simulink model "AFS_Master"  (R2020b)
settings: configuration reference "VLS_Standard_Configuration" (kept outside this file)
undefined symbols (not defined in the file): C_AFS_SpeedThrAct
libraries: AFS_MasterFeature x2
settings Model: DataDictionary=AFS_Master_Model.sldd  Creator=mmoufakk  LastModifiedBy=mtarek-a
settings ConfigSetRef: SourceName=VLS_Standard_Configuration

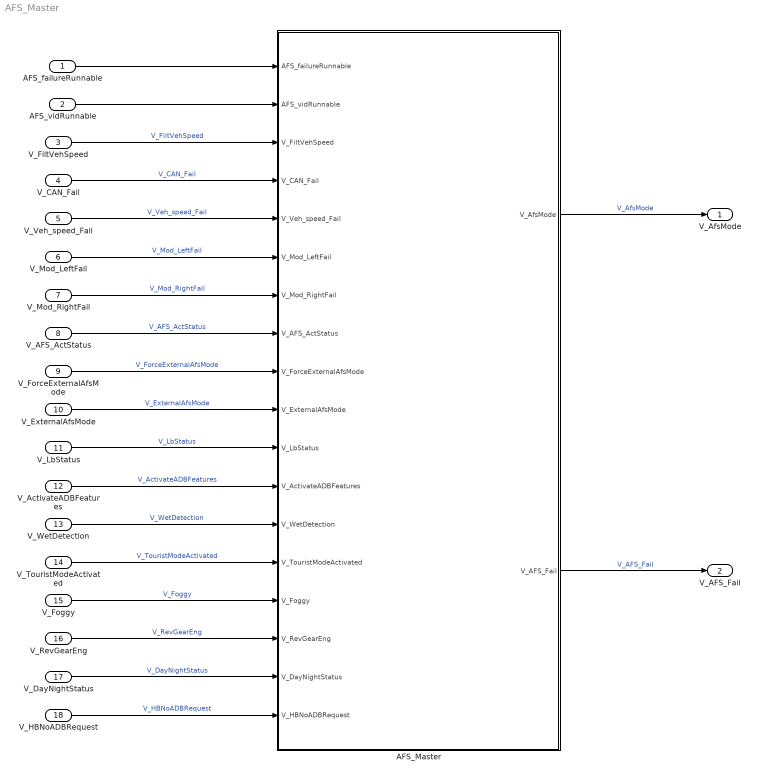
== system AFS_Master ==
  AFS_failureRunnable : Inport  OutputFunctionCall=on
  AFS_vidRunnable : Inport  Port=2  OutputFunctionCall=on
  V_FiltVehSpeed : Inport  Port=3
  V_CAN_Fail : Inport  Port=4
  V_Veh_speed_Fail : Inport  Port=5
  V_Mod_LeftFail : Inport  Port=6
  V_Mod_RightFail : Inport  Port=7
  V_AFS_ActStatus : Inport  Port=8
  V_ForceExternalAfsMode : Inport  Port=9
  V_ExternalAfsMode : Inport  Port=10
  V_LbStatus : Inport  Port=11
  V_ActivateADBFeatures : Inport  Port=12
  V_WetDetection : Inport  Port=13
  V_TouristModeActivated : Inport  Port=14
  V_Foggy : Inport  Port=15
  V_RevGearEng : Inport  Port=16
  V_DayNightStatus : Inport  Port=17
  V_HBNoADBRequest : Inport  Port=18
  AFS_Master : Subsystem  Description=AFS_Master
  V_AfsMode : Outport  PortDimensions=1
  V_AFS_Fail : Outport  Port=2  VectorParamsAs1DForOutWhenUnconnected=off
  wires:
  AFS_Master/1(V_AfsMode) -> V_AfsMode/1  "V_AfsMode"
  AFS_Master/2(V_AFS_Fail) -> V_AFS_Fail/1  "V_AFS_Fail"
  AFS_failureRunnable/1 -> AFS_Master/1(AFS_failureRunnable)
  AFS_vidRunnable/1 -> AFS_Master/2(AFS_vidRunnable)
  V_CAN_Fail/1 -> AFS_Master/4(V_CAN_Fail)  "V_CAN_Fail"
  V_Veh_speed_Fail/1 -> AFS_Master/5(V_Veh_speed_Fail)  "V_Veh_speed_Fail"
  V_Mod_LeftFail/1 -> AFS_Master/6(V_Mod_LeftFail)  "V_Mod_LeftFail"
  V_FiltVehSpeed/1 -> AFS_Master/3(V_FiltVehSpeed)  "V_FiltVehSpeed"
  V_ActivateADBFeatures/1 -> AFS_Master/12(V_ActivateADBFeatures)  "V_ActivateADBFeatures"
  V_Mod_RightFail/1 -> AFS_Master/7(V_Mod_RightFail)  "V_Mod_RightFail"
  V_AFS_ActStatus/1 -> AFS_Master/8(V_AFS_ActStatus)  "V_AFS_ActStatus"
  V_LbStatus/1 -> AFS_Master/11(V_LbStatus)  "V_LbStatus"
  V_WetDetection/1 -> AFS_Master/13(V_WetDetection)  "V_WetDetection"
  V_TouristModeActivated/1 -> AFS_Master/14(V_TouristModeActivated)  "V_TouristModeActivated"
  V_Foggy/1 -> AFS_Master/15(V_Foggy)  "V_Foggy"
  V_RevGearEng/1 -> AFS_Master/16(V_RevGearEng)  "V_RevGearEng"
  V_DayNightStatus/1 -> AFS_Master/17(V_DayNightStatus)  "V_DayNightStatus"
  V_HBNoADBRequest/1 -> AFS_Master/18(V_HBNoADBRequest)  "V_HBNoADBRequest"
  V_ForceExternalAfsMode/1 -> AFS_Master/9(V_ForceExternalAfsMode)  "V_ForceExternalAfsMode"
  V_ExternalAfsMode/1 -> AFS_Master/10(V_ExternalAfsMode)  "V_ExternalAfsMode"

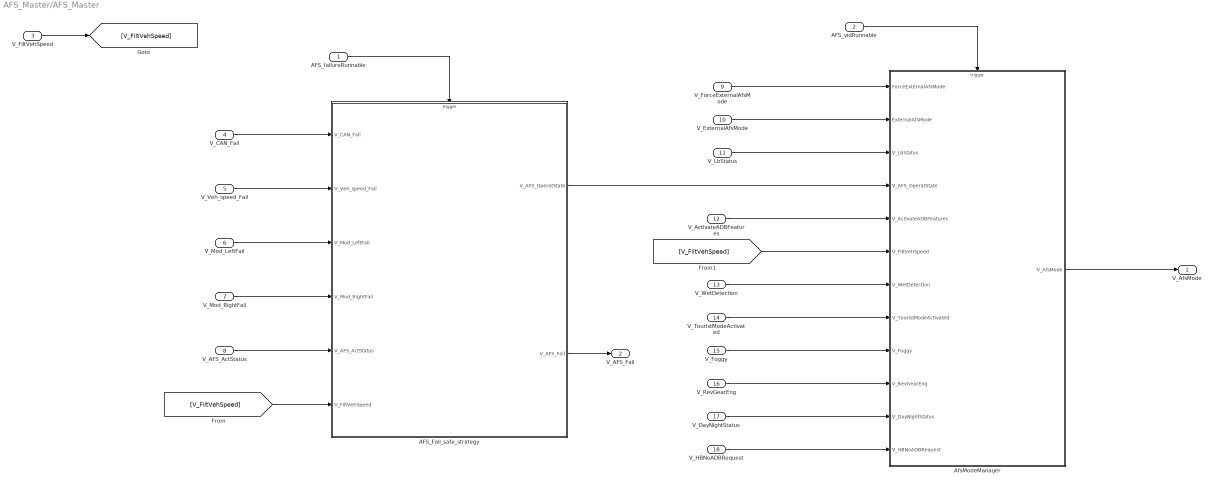
== system AFS_Master/AFS_Master ==
  AFS_failureRunnable : Inport  OutputFunctionCall=on
  AFS_vidRunnable : Inport  Port=2  OutputFunctionCall=on
  V_FiltVehSpeed : Inport  Port=3
  V_CAN_Fail : Inport  Port=4
  V_Veh_speed_Fail : Inport  Port=5
  V_Mod_LeftFail : Inport  Port=6
  V_Mod_RightFail : Inport  Port=7
  V_AFS_ActStatus : Inport  Port=8
  V_ForceExternalAfsMode : Inport  Port=9
  V_ExternalAfsMode : Inport  Port=10
  V_LbStatus : Inport  Port=11
  V_ActivateADBFeatures : Inport  Port=12
  V_WetDetection : Inport  Port=13
  V_TouristModeActivated : Inport  Port=14
  V_Foggy : Inport  Port=15
  V_RevGearEng : Inport  Port=16
  V_DayNightStatus : Inport  Port=17
  V_HBNoADBRequest : Inport  Port=18
  AFS_Fail_safe_strategy : Subsystem  Description=AFS_Fail_safe_strategy
  AfsModeManager : Subsystem  Description=AfsModeManager
  V_AfsMode : Outport  PortDimensions=1
  V_AFS_Fail : Outport  Port=2  VectorParamsAs1DForOutWhenUnconnected=off
  wires:
  V_HBNoADBRequest/1 -> AfsModeManager/12(V_HBNoADBRequest)
  V_DayNightStatus/1 -> AfsModeManager/11(V_DayNightStatus)
  AFS_Fail_safe_strategy/1(V_AFS_OperatState) -> AfsModeManager/4(V_AFS_OperatState)
  V_Mod_RightFail/1 -> AFS_Fail_safe_strategy/4(V_Mod_RightFail)
  V_Mod_LeftFail/1 -> AFS_Fail_safe_strategy/3(V_Mod_LeftFail)
  AFS_Fail_safe_strategy/2(V_AFS_Fail) -> V_AFS_Fail/1
  [V_FiltVehSpeed] -> AfsModeManager/6(V_FiltVehSpeed)
  [V_FiltVehSpeed] -> AFS_Fail_safe_strategy/6(V_FiltVehSpeed)
  V_FiltVehSpeed/1 -> [V_FiltVehSpeed]
  V_AFS_ActStatus/1 -> AFS_Fail_safe_strategy/5(V_AFS_ActStatus)
  AFS_failureRunnable/1 -> AFS_Fail_safe_strategy/Trigger
  V_Veh_speed_Fail/1 -> AFS_Fail_safe_strategy/2(V_Veh_speed_Fail)
  V_CAN_Fail/1 -> AFS_Fail_safe_strategy/1(V_CAN_Fail)
  AFS_vidRunnable/1 -> AfsModeManager/Trigger
  V_Foggy/1 -> AfsModeManager/9(V_Foggy)
  V_ForceExternalAfsMode/1 -> AfsModeManager/1(ForceExternalAfsMode)
  V_LbStatus/1 -> AfsModeManager/3(V_LbStatus)
  V_WetDetection/1 -> AfsModeManager/7(V_WetDetection)
  AfsModeManager/1(V_AfsMode) -> V_AfsMode/1
  V_RevGearEng/1 -> AfsModeManager/10(V_RevGearEng)
  V_ExternalAfsMode/1 -> AfsModeManager/2(ExternalAfsMode)
  V_ActivateADBFeatures/1 -> AfsModeManager/5(V_ActivateADBFeatures)
  V_TouristModeActivated/1 -> AfsModeManager/8(V_TouristModeActivated)

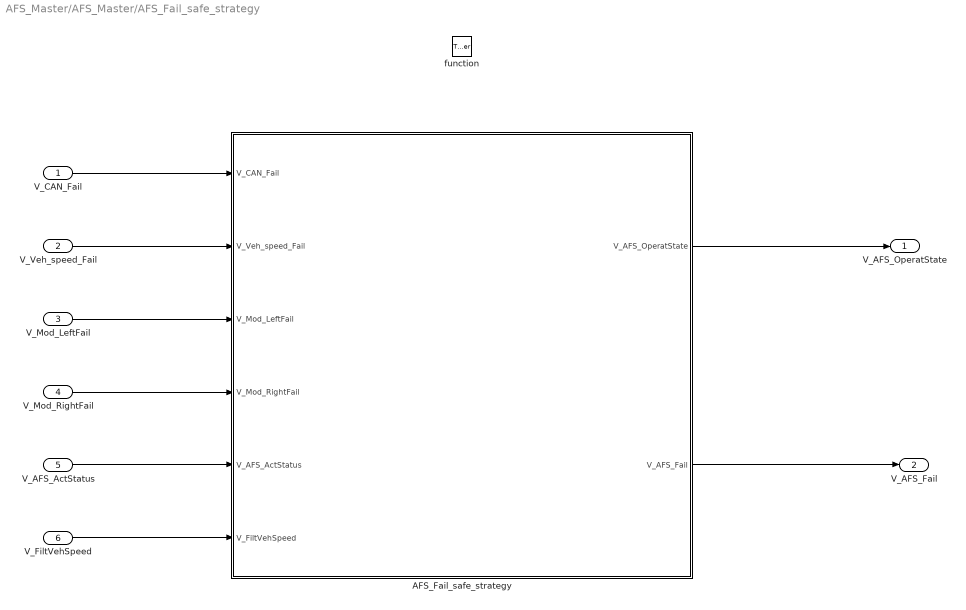
== system AFS_Master/AFS_Master/AFS_Fail_safe_strategy ==
  V_CAN_Fail : Inport
  V_Veh_speed_Fail : Inport  Port=2
  V_Mod_LeftFail : Inport  Port=3
  V_Mod_RightFail : Inport  Port=4
  V_AFS_ActStatus : Inport  Port=5
  V_FiltVehSpeed : Inport  Port=6
  function : TriggerPort  TriggerType=function-call  VariantControl=Variant
  AFS_Fail_safe_strategy : Subsystem  Description=AFS_Fail_safe_strategy
  V_AFS_OperatState : Outport  VectorParamsAs1DForOutWhenUnconnected=off
  V_AFS_Fail : Outport  Port=2  VectorParamsAs1DForOutWhenUnconnected=off
  wires:
  V_Veh_speed_Fail/1 -> AFS_Fail_safe_strategy/2(V_Veh_speed_Fail)
  V_CAN_Fail/1 -> AFS_Fail_safe_strategy/1(V_CAN_Fail)
  V_AFS_ActStatus/1 -> AFS_Fail_safe_strategy/5(V_AFS_ActStatus)
  V_Mod_LeftFail/1 -> AFS_Fail_safe_strategy/3(V_Mod_LeftFail)
  V_Mod_RightFail/1 -> AFS_Fail_safe_strategy/4(V_Mod_RightFail)
  AFS_Fail_safe_strategy/2(V_AFS_Fail) -> V_AFS_Fail/1
  AFS_Fail_safe_strategy/1(V_AFS_OperatState) -> V_AFS_OperatState/1
  V_FiltVehSpeed/1 -> AFS_Fail_safe_strategy/6(V_FiltVehSpeed)

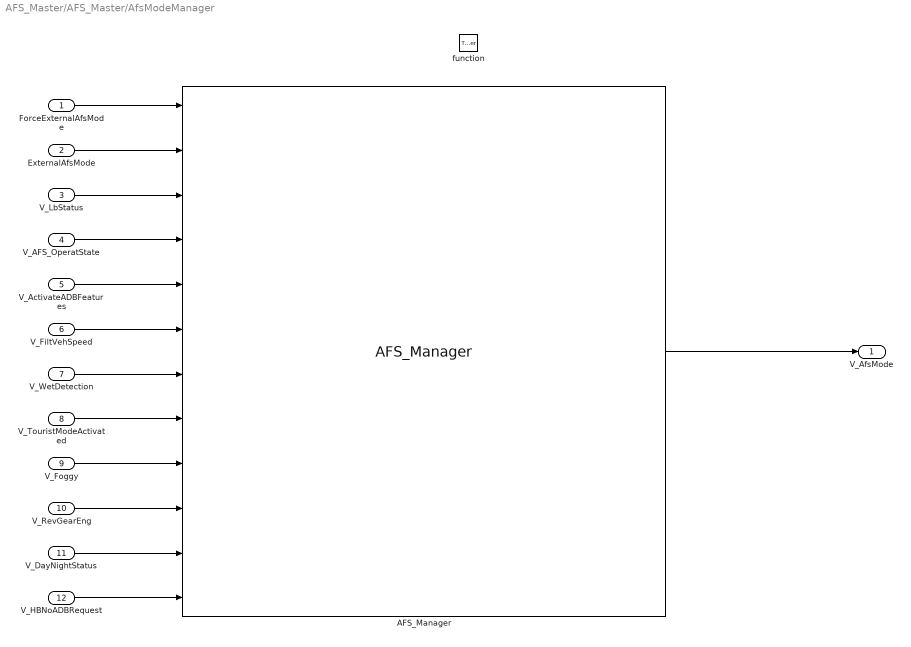
== system AFS_Master/AFS_Master/AfsModeManager ==
  ForceExternalAfsMode : Inport
  ExternalAfsMode : Inport  Port=2
  V_LbStatus : Inport  Port=3
  V_AFS_OperatState : Inport  Port=4
  V_ActivateADBFeatures : Inport  Port=5
  V_FiltVehSpeed : Inport  Port=6
  V_WetDetection : Inport  Port=7
  V_TouristModeActivated : Inport  Port=8
  V_Foggy : Inport  Port=9
  V_RevGearEng : Inport  Port=10
  V_DayNightStatus : Inport  Port=11
  V_HBNoADBRequest : Inport  Port=12
  function : TriggerPort  TriggerType=function-call  VariantControl=Variant
  AFS_Manager : AFS_MasterFeature/AFS_Manager  Description=AFS_Subsystem  SystemSampleTime=-1  VariantActivationTime=update diagram  Latency=0  AutoFrameSizeCalculation=off
  V_AfsMode : Outport  PortDimensions=1
  wires:
  ExternalAfsMode/1 -> AFS_Manager/2
  ForceExternalAfsMode/1 -> AFS_Manager/1
  V_LbStatus/1 -> AFS_Manager/3
  V_ActivateADBFeatures/1 -> AFS_Manager/5
  V_FiltVehSpeed/1 -> AFS_Manager/6
  V_WetDetection/1 -> AFS_Manager/7
  V_TouristModeActivated/1 -> AFS_Manager/8
  V_Foggy/1 -> AFS_Manager/9
  AFS_Manager/1 -> V_AfsMode/1
  V_RevGearEng/1 -> AFS_Manager/10
  V_AFS_OperatState/1 -> AFS_Manager/4
  V_DayNightStatus/1 -> AFS_Manager/11
  V_HBNoADBRequest/1 -> AFS_Manager/12

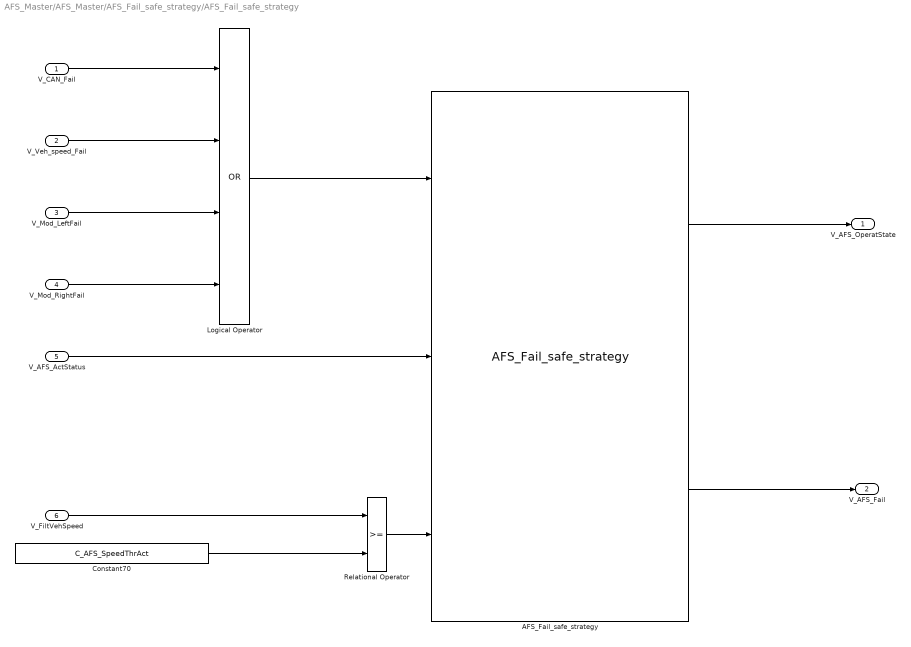
== system AFS_Master/AFS_Master/AFS_Fail_safe_strategy/AFS_Fail_safe_strategy ==
  V_CAN_Fail : Inport
  V_Veh_speed_Fail : Inport  Port=2
  V_Mod_LeftFail : Inport  Port=3
  V_Mod_RightFail : Inport  Port=4
  V_AFS_ActStatus : Inport  Port=5
  V_FiltVehSpeed : Inport  Port=6
  AFS_Fail_safe_strategy : AFS_MasterFeature/AFS_Fail_safe_strategy  Description=AFS_Fail_safe_strategy  SystemSampleTime=-1  VariantActivationTime=update diagram  Latency=0  AutoFrameSizeCalculation=off
  Constant70 : Constant  Value=C_AFS_SpeedThrAct
  Logical Operator : Logic  Operator=OR  Inputs=4  AllPortsSameDT=off  OutDataTypeStr=boolean
  Relational Operator : RelationalOperator  OutDataTypeStr=boolean
  V_AFS_OperatState : Outport  VectorParamsAs1DForOutWhenUnconnected=off
  V_AFS_Fail : Outport  Port=2  VectorParamsAs1DForOutWhenUnconnected=off
  wires:
  V_Mod_RightFail/1 -> Logical Operator/4
  V_AFS_ActStatus/1 -> AFS_Fail_safe_strategy/2
  V_CAN_Fail/1 -> Logical Operator/1
  V_Veh_speed_Fail/1 -> Logical Operator/2
  V_Mod_LeftFail/1 -> Logical Operator/3
  V_FiltVehSpeed/1 -> Relational Operator/1
  Logical Operator/1 -> AFS_Fail_safe_strategy/1
  Constant70/1 -> Relational Operator/2
  AFS_Fail_safe_strategy/2 -> V_AFS_Fail/1
  Relational Operator/1 -> AFS_Fail_safe_strategy/3
  AFS_Fail_safe_strategy/1 -> V_AFS_OperatState/1
